simulink model "traffic_light_simulation"  (R2014a)
settings: Solver=FixedStepDiscrete  StartTime=0.0  StopTime=inf  FixedStep=0.02  RelTol=1e-3
model workspace (MAT data in the model file):
  Te = 0.1
CloseFcn:
  | rtwprivate ssgencode ModelCloseRequest traffic_light
settings Model: ExtModeTrigDuration=2  Creator=deastman  LastModifiedBy=ningd
settings OptimizationCC: ExpressionDepthLimit=2147483647  OptimizeModelRefInitCode=on  LifeSpan=Inf
settings DebuggingCC: UnderspecifiedInitializationDetection=Classic  StateNameClashWarn=warning
settings HardwareCC: ProdLargestAtomicInteger=Integer  ProdLargestAtomicFloat=Float  ProdIntDivRoundTo=Zero  ProdEndianess=LittleEndian  ProdHWDeviceType=STMicroelectronics->STM32F4xx 32-bit Cortex-M4
settings RTWCC: SystemTargetFile=ert.tlc  GenCodeOnly=on  TemplateMakefile=ert_default_tmf  Description=Embedded Coder  GenerateReport=on  ProcessScript=ert_make_rtw_hook  IncludeHyperlinkInReport=on  LaunchReport=on  GenerateTraceInfo=on  GenerateTraceReport=on  GenerateTraceReportSl=on  GenerateTraceReportSf=on  GenerateTraceReportEml=on
settings CodeAppCC: IgnoreCustomStorageClasses=off  CustomSymbolStrType=$N$R$M  InternalIdentifier=Classic
settings ERTTargetCC: ParMdlRefBuildCompliant=on  CompOptLevelCompliant=on  ConcurrentExecutionCompliant=on  ERTFirstTimeCompliant=on  ModelStepFunctionPrototypeControlCompliant=on  CPPClassGenCompliant=on  InlinedParameterPlacement=Hierarchical  ERTCustomFileTemplate=example_file_process.tlc

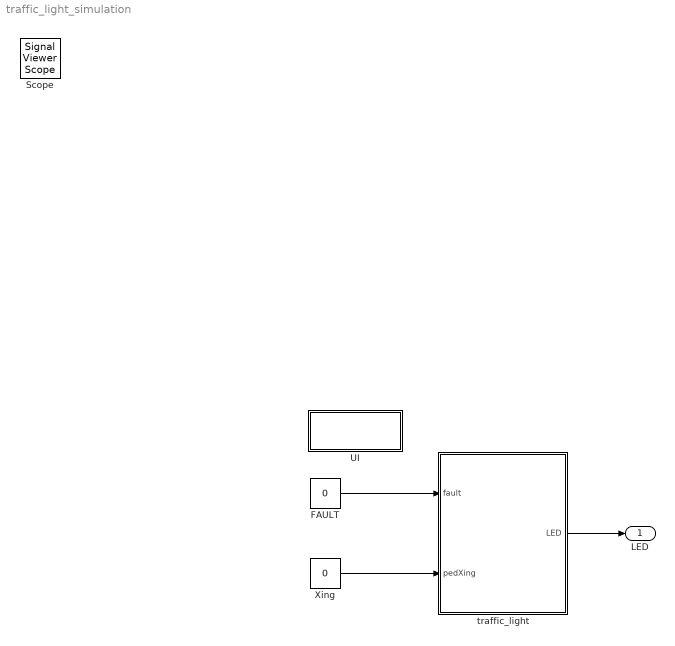
== system traffic_light_simulation ==
  FAULT : Constant  Value=0  OutDataTypeStr=boolean
  UI : Subsystem
      mask DialogControl Container1 Prompt: Buttons
      mask Display: image('UI.png')
  Xing : Constant  Value=0  OutDataTypeStr=boolean
  traffic_light : Subsystem
  LED : Outport
  Scope : SignalViewerScope  IOType=viewer  RefreshTime=0.035000
  wires:
  traffic_light/1(LED) -> LED/1
  FAULT/1 -> traffic_light/1(fault)
  Xing/1 -> traffic_light/2(pedXing)

== system traffic_light_simulation/UI ==

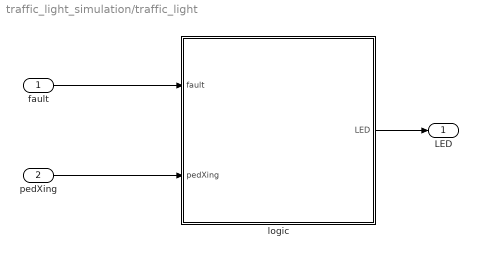
== system traffic_light_simulation/traffic_light ==
  fault : Inport
  pedXing : Inport  Port=2
  logic : Stateflow chart  TreatAsAtomicUnit=on
  LED : Outport
  wires:
  fault/1 -> logic/1(fault)
  logic/1(LED) -> LED/1
  pedXing/1 -> logic/2(pedXing)

== stateflow chart traffic_light_simulation/traffic_light/logic ==
  state Normal
    (history)
    state LIGHT_RED
      en : LED = RED;
    state LIGHT_ORANGE
      en : LED = ORANGE;
    state LIGHT_GREEN
      en : LED = GREEN;
    (default) -> LIGHT_RED
    LIGHT_ORANGE -> LIGHT_RED : after(2/Ts,tick)
    LIGHT_RED -> LIGHT_GREEN : after(5/Ts,tick)
    LIGHT_GREEN -> LIGHT_ORANGE [order 1] : [pedXing]
    LIGHT_GREEN -> LIGHT_ORANGE [order 2] : [after(5/Ts,tick)]
  state flash_LED [function]
    (default) -> (junction 44) : /* Blink */
    (junction 44) -> (junction 43) [order 1] : [LED == ORANGE]
    (junction 44) -> (junction 45) [order 2] : {LED = ORANGE;}
    (junction 43) -> (junction 42) : {LED = OFF;}
    (junction 42) -> (junction 45)
    (junction 45) -> (junction 41)
  state Faulty
    en : flash_LED()
  (default) -> Normal
  Normal -> Faulty : [fault]
  Faulty -> Normal [order 1] : [!fault]
  Faulty -> Faulty [order 2] : after(1/Ts,tick)
  data: LED output double; OFF constant double =0; fault input; GREEN local double =1; ORANGE local double =2; RED local double =3; pedXing input; Ts constant double =Te
